simulink model "problem5_sim"  (R2024a)
settings: Solver=VariableStepAuto  StartTime=0.0  StopTime=10.0  RelTol=1e-3
undefined symbols (not defined in the file): A, B, C, D, F, K, L, u_amp, u_w, useSine
settings Model: Creator=dunni  LastModifiedBy=dunni

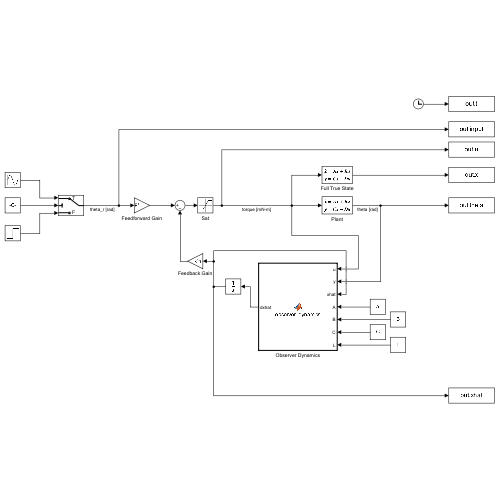
[thumbnail: Simulink's stored preview of the top-level diagram]
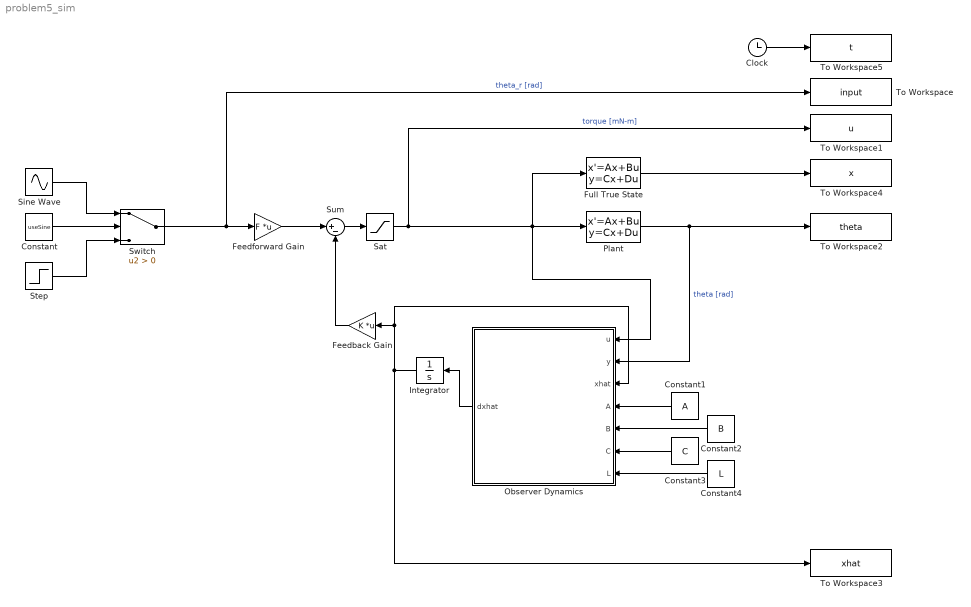
== system problem5_sim ==
  Clock : Clock
  Constant : Constant  Value=useSine
  Constant1 : Constant  Value=A  VectorParams1D=off
  Constant2 : Constant  Value=B  VectorParams1D=off
  Constant3 : Constant  Value=C  VectorParams1D=off
  Constant4 : Constant  Value=L  VectorParams1D=off
  Feedback Gain : Gain  Gain=K  Multiplication=Matrix(K*u)
  Feedforward Gain : Gain  Gain=F  Multiplication=Matrix(K*u)
  Full True State : StateSpace  A=A  B=B  C=eye(4)  D=zeros(4,1)  InitialCondition=0
  Integrator : Integrator  InitialCondition=[0.1; 0.1; 0.1; 0.1]
  Observer Dynamics : MATLAB Function  TreatAsAtomicUnit=on
  Plant : StateSpace  A=A  B=B  C=C  D=D  InitialCondition=0
  Sat : Saturate  UpperLimit=67  LowerLimit=-67
  Sine Wave : Sin  Amplitude=u_amp  Frequency=u_w  SampleTime=0
  Step : Step  After=u_amp  SampleTime=0
  Sum : Sum  Inputs=|+-
  Switch : Switch  Criteria=u2 > Threshold  SaturateOnIntegerOverflow=off  InputSameDT=off
  To Workspace : ToWorkspace  VariableName=input  SaveFormat=Timeseries  SampleTime=-1
  To Workspace1 : ToWorkspace  VariableName=u  SaveFormat=Timeseries  SampleTime=-1
  To Workspace2 : ToWorkspace  VariableName=theta  SaveFormat=Timeseries  SampleTime=-1
  To Workspace3 : ToWorkspace  VariableName=xhat  SampleTime=-1
  To Workspace4 : ToWorkspace  VariableName=x  SampleTime=-1
  To Workspace5 : ToWorkspace  VariableName=t  SampleTime=-1
  wires:
  Constant/1 -> Switch/2
  Sine Wave/1 -> Switch/1
  Step/1 -> Switch/3
  Switch/1 -> To Workspace/1, Feedforward Gain/1  "theta_r [rad]"
  Feedforward Gain/1 -> Sum/1
  Feedback Gain/1 -> Sum/2
  Sum/1 -> Sat/1
  Sat/1 -> To Workspace1/1, Full True State/1, Observer Dynamics/1(u), Plant/1  "torque [mN-m]"
  Plant/1 -> Observer Dynamics/2(y), To Workspace2/1  "theta [rad]"
  Observer Dynamics/1(dxhat) -> Integrator/1
  Integrator/1 -> To Workspace3/1, Feedback Gain/1, Observer Dynamics/3(xhat)
  Constant1/1 -> Observer Dynamics/4(A)
  Constant2/1 -> Observer Dynamics/5(B)
  Constant3/1 -> Observer Dynamics/6(C)
  Constant4/1 -> Observer Dynamics/7(L)
  Full True State/1 -> To Workspace4/1
  Clock/1 -> To Workspace5/1

== matlab function problem5_sim/Observer Dynamics ==
  data: u input; dxhat output; y input; xhat input; A input; B input; C input; L input
function dxhat = observer_dynamics(u, y, xhat, A, B, C, L)
% Takes as input the control input u, the measured state y, and the current
% state xhat
% Outputs the rate of change of the state xhat
% Inputs:
%   u -> control input
%   y -> measured output
%   xhat -> current estimated state
%   const_struct -> A, B, C, L matrices for observer dynamics
% Outputs:
%   dxhat -> Rate of change of estimated state


dxhat = (A - L*C)*xhat + B*u + L*y;
